simulink model "Model0_PWM_Base"  (R2021b)
settings: Solver=ode23s  StartTime=0.0  StopTime=20  MaxStep=1e-6  RelTol=1e-5  EnableMultiTasking=on
InitFcn:
  | L=5e-3
  | R=0.1
  | tau=10e-3
  | f_grid=50
  | Vpeak_d1=400*sqrt(2)/sqrt(3)
libraries: spsIGBTDiodeLib x6, spsControlledVoltageSourceLib x3, spsCurrentMeasurementLib x3, spsSeriesRLCBranchLib x3, spsVoltageMeasurementLib x3, spsDCVoltageSourceLib x2, spsGroundLib x1, simulink x1, spspowerguiLib x1
settings Model: Creator=Eduardo  LastModifiedBy=eprieto
settings SolverCC: ZeroCrossAlgorithm=Adaptive  AlgebraicLoopSolver=TrustRegion
settings DataIOCC: LimitDataPoints=on  SaveFormat=Array  SignalLoggingSaveFormat=ModelDataLogs  ReturnWorkspaceOutputs=off
settings OptimizationCC: LifeSpan=inf
settings DebuggingCC: SolverPrmCheckMsg=warning  MultiTaskDSMMsg=warning  MultiTaskCondExecSysMsg=none  StrictBusMsg=ErrorOnBusTreatedAsVector  SFUnexpectedBacktrackingDiag=warning  SFNoUnconditionalDefaultTransitionDiag=warning  SFExecutionAtInitializationDiag=none  SFMachineParentedDataDiag=warning  ArithmeticOperatorsInVariantConditions=warning
settings HardwareCC: ProdBitPerPointer=32  ProdBitPerSizeT=32  ProdBitPerPtrDiffT=32  ProdLargestAtomicFloat=None  ProdIntDivRoundTo=Undefined  ProdEndianess=Unspecified  ProdWordSize=32  ProdHWDeviceType=32-bit Generic
settings ModelReferenceCC: PropagateSignalLabelsOutOfModel=off
settings SFSimCC: SimUseLocalCustomCode=off  CustomCodeUndefinedFunction=UseInterfaceOnly
settings RTWCC: RTWUseLocalCustomCode=off
settings CodeAppCC: StateflowObjectComments=on
settings GRTTargetCC: TargetLangStandard=C89/C90 (ANSI)
settings ConfigComp: CovMetricSettings=dw  CovSaveCumulativeToWorkspaceVar=on  CovSaveSingleToWorkspaceVar=on  CovExternalEMLEnable=off
settings SimscapeCC: SimscapeNormalizeSystem=off

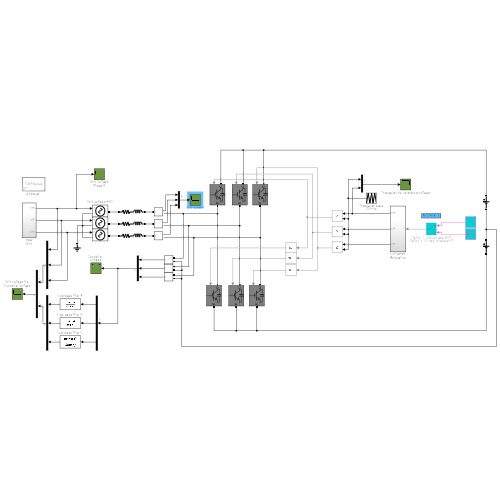
[thumbnail: Simulink's stored preview of the top-level diagram]
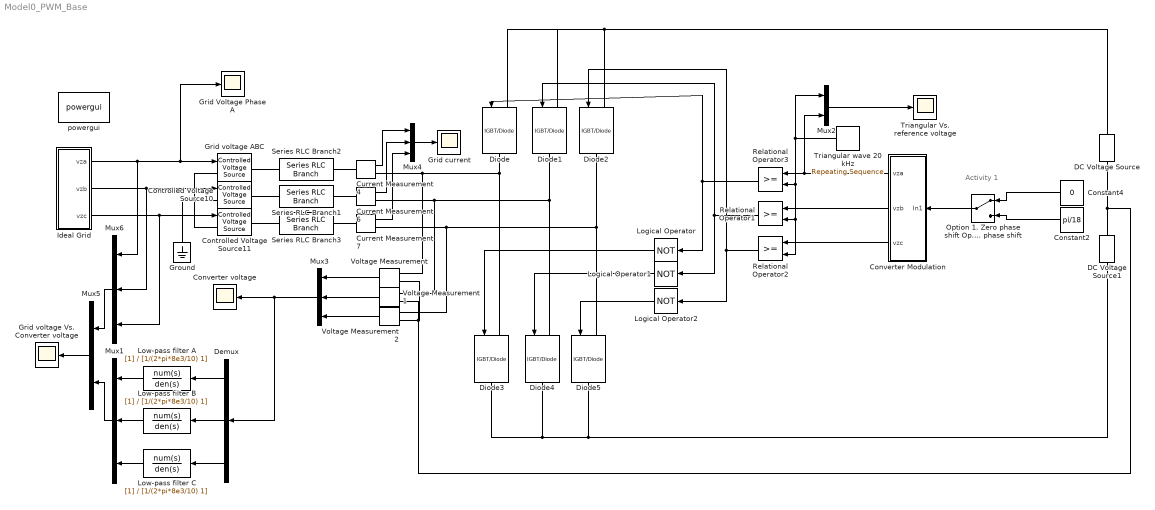
== system Model0_PWM_Base ==
  note: Activity 1
  Constant2 : Constant  Value=pi/18
  Constant4 : Constant  Value=0
  Controlled Voltage Source10 : spsControlledVoltageSourceLib/Controlled Voltage Source  Initialize=off  Source_Type=AC  Amplitude=0  Phase=0  Frequency=0  Measurements=None
  Controlled Voltage Source11 : spsControlledVoltageSourceLib/Controlled Voltage Source  Initialize=off  Source_Type=AC  Amplitude=0  Phase=0  Frequency=0  Measurements=None
  Converter Modulation : Subsystem
  Converter voltage : Scope
  Current Measurement4 : spsCurrentMeasurementLib/Current Measurement  PhasorSimulation=off  OutputType=Complex  PSBequivalent=0
  Current Measurement6 : spsCurrentMeasurementLib/Current Measurement  PhasorSimulation=off  OutputType=Complex  PSBequivalent=0
  Current Measurement7 : spsCurrentMeasurementLib/Current Measurement  PhasorSimulation=off  OutputType=Complex  PSBequivalent=0
  DC Voltage Source : spsDCVoltageSourceLib/DC Voltage Source  Amplitude=Vpeak_d1  Measurements=None
  DC Voltage Source1 : spsDCVoltageSourceLib/DC Voltage Source  Amplitude=Vpeak_d1  Measurements=None
  Demux : Demux  Outputs=3
  Diode{,1..5} (6 alike) : spsIGBTDiodeLib/IGBT//Diode  Ron=1e-3  Rs=1e5  Cs=inf  Measurements=off
  Grid Voltage Phase A : Scope
  Grid current : Scope
  Grid voltage ABC : spsControlledVoltageSourceLib/Controlled Voltage Source  Initialize=off  Source_Type=AC  Amplitude=0  Phase=0  Frequency=0  Measurements=None
  Grid voltage Vs. Converter voltage : Scope
  Ground : spsGroundLib/Ground  LConnTagsString=a
  Ideal Grid : Subsystem
  Logical Operator : Logic  Operator=NOT  AllPortsSameDT=off
  Logical Operator1 : Logic  Operator=NOT  AllPortsSameDT=off
  Logical Operator2 : Logic  Operator=NOT  AllPortsSameDT=off
  Low-pass filter A : TransferFcn  Denominator=[1/(2*pi*8e3/10) 1]
  Low-pass filter B : TransferFcn  Denominator=[1/(2*pi*8e3/10) 1]
  Low-pass filter C : TransferFcn  Denominator=[1/(2*pi*8e3/10) 1]
  Mux{1,3..4,6} (4 alike) : Mux  Inputs=3
  Mux2 : Mux  Inputs=2
  Mux5 : Mux  Inputs=2
  "Option 1. Zero phase shift Option 2. 20 deg. phase shift " : ManualSwitch
  Relational Operator1 : RelationalOperator  RndMeth=Nearest
  Relational Operator2 : RelationalOperator  RndMeth=Nearest
  Relational Operator3 : RelationalOperator  RndMeth=Nearest
  Series RLC Branch1 : spsSeriesRLCBranchLib/Series RLC Branch  LConnTagsString=__new0  RConnTagsString=__new0  BranchType=RL  Resistance=R  Inductance=L  SetiL0=off  InitialCurrent=0  Capacitance=0  Setx0=off  InitialVoltage=0  Measurements=None
  Series RLC Branch2 : spsSeriesRLCBranchLib/Series RLC Branch  LConnTagsString=__new0  RConnTagsString=__new0  BranchType=RL  Resistance=R  Inductance=L  SetiL0=off  InitialCurrent=0  Capacitance=0  Setx0=off  InitialVoltage=0  Measurements=None
  Series RLC Branch3 : spsSeriesRLCBranchLib/Series RLC Branch  LConnTagsString=__new0  RConnTagsString=__new0  BranchType=RL  Resistance=R  Inductance=L  SetiL0=off  InitialCurrent=0  Capacitance=0  Setx0=off  InitialVoltage=0  Measurements=None
  Triangular Vs. reference voltage : Scope
  Triangular wave 20 kHz : simulink/Sources/Repeating Sequence  rep_seq_t=[0 1/20e3 1/20e3*2]  rep_seq_y=[-Vpeak_d1 Vpeak_d1 -Vpeak_d1]
  Voltage Measurement : spsVoltageMeasurementLib/Voltage Measurement  PhasorSimulation=off  OutputType=Complex  PSBequivalent=0
  Voltage Measurement1 : spsVoltageMeasurementLib/Voltage Measurement  PhasorSimulation=off  OutputType=Complex  PSBequivalent=0
  Voltage Measurement2 : spsVoltageMeasurementLib/Voltage Measurement  PhasorSimulation=off  OutputType=Complex  PSBequivalent=0
  powergui : spspowerguiLib/powergui  Priority=1  SimulationMode=Continuous  SampleTime=50e-6  frequency=60  Iterations=50  frequencyindice=0  Pbase=100e6  ErrMax=1e-4  UnitsV=kV  UnitsW=MW  buscounter=0  FunctionMessages=off  echomessages=off  EnableUseOfTLC=off  CurrentSourceSwitches=off  DisableSnubberDevices=off  DisableRonSwitches=off  DisableVfSwitches=off  DisplayEquations=off  AutomaticDiscreteSolvers=off  SolverType=Tustin  Interpol=off  ExternalGateDelay=off  methode=off  Ts=0  x0status=blocks  SPID=off  SwTol=0  HookPort=off  NonlinearTolerance=1e-4  nMaxIteration=100  ContinueOnMaxIteration=off  RestoreLinks=warning  ResistiveCurrentMeasurement=off  Frange=[0:2:500]  Ylog=off  Xlog=on  ShowGrid=off  save=off  variable=ZData  structure=0  ZoomFFT=off  StartTime=0.0  cycles=1  DisplayStyle=1  fundamental=60  FreqAxis=off  MaxFrequency=1000  frequencyindicesteady=1  RmsSteady=1  display=off
  wires:
  Ideal Grid/1(vza) -> Mux6/1, Grid Voltage Phase A/1, Grid voltage ABC/1
  Ideal Grid/2(vzb) -> Mux6/2, Controlled Voltage Source10/1
  Ideal Grid/3(vzc) -> Mux6/3, Controlled Voltage Source11/1
  Current Measurement4/1 -> Mux4/1
  Current Measurement6/1 -> Mux4/2
  Current Measurement7/1 -> Mux4/3
  Converter Modulation/1(vza) -> Relational Operator3/1, Mux2/2
  Converter Modulation/2(vzb) -> Relational Operator1/1
  Converter Modulation/3(vzc) -> Relational Operator2/1
  Relational Operator3/1 -> Diode/1, Logical Operator/1
  Relational Operator1/1 -> Diode1/1, Logical Operator1/1
  Relational Operator2/1 -> Diode2/1, Logical Operator2/1
  Logical Operator/1 -> Diode3/1
  Mux2/1 -> Triangular Vs. reference voltage/1
  Voltage Measurement/1 -> Mux3/1
  Voltage Measurement1/1 -> Mux3/2
  Mux3/1 -> Converter voltage/1, Demux/1
  Mux4/1 -> Grid current/1
  Logical Operator1/1 -> Diode4/1
  Logical Operator2/1 -> Diode5/1
  Constant4/1 -> "Option 1. Zero phase shift Option 2. 20 deg. phase shift "/1
  Constant2/1 -> "Option 1. Zero phase shift Option 2. 20 deg. phase shift "/2
  "Option 1. Zero phase shift Option 2. 20 deg. phase shift "/1 -> Converter Modulation/1(In1)
  Voltage Measurement2/1 -> Mux3/3
  Triangular wave 20 kHz/1 -> Relational Operator3/2, Relational Operator2/2, Relational Operator1/2, Mux2/1
  Demux/1 -> Low-pass filter A/1
  Demux/2 -> Low-pass filter B/1
  Demux/3 -> Low-pass filter C/1
  Low-pass filter C/1 -> Mux1/3
  Low-pass filter B/1 -> Mux1/2
  Low-pass filter A/1 -> Mux1/1
  Mux5/1 -> Grid voltage Vs. Converter voltage/1
  Mux1/1 -> Mux5/2
  Mux6/1 -> Mux5/1
  connections:
  Grid voltage ABC/LConn1 -- Ground/LConn1 -- Controlled Voltage Source10/LConn1 -- Controlled Voltage Source11/LConn1
  Current Measurement6/RConn1 -- Voltage Measurement1/LConn1 -- Diode1/RConn1 -- Diode4/LConn1
  Current Measurement4/LConn1 -- Series RLC Branch2/RConn1
  Series RLC Branch2/LConn1 -- Grid voltage ABC/RConn1
  Current Measurement7/LConn1 -- Series RLC Branch3/RConn1
  Current Measurement6/LConn1 -- Series RLC Branch1/RConn1
  Series RLC Branch3/LConn1 -- Controlled Voltage Source11/RConn1
  Current Measurement4/RConn1 -- Voltage Measurement/LConn1 -- Diode3/LConn1 -- Diode/RConn1
  Series RLC Branch1/LConn1 -- Controlled Voltage Source10/RConn1
  Diode1/LConn1 -- Diode/LConn1 -- DC Voltage Source/RConn1 -- Diode2/LConn1
  Diode3/RConn1 -- DC Voltage Source1/LConn1 -- Diode5/RConn1 -- Diode4/RConn1
  Current Measurement7/RConn1 -- Voltage Measurement2/LConn1 -- Diode2/RConn1 -- Diode5/LConn1
  DC Voltage Source/LConn1 -- Voltage Measurement2/LConn2 -- Voltage Measurement/LConn2 -- Voltage Measurement1/LConn2 -- DC Voltage Source1/RConn1

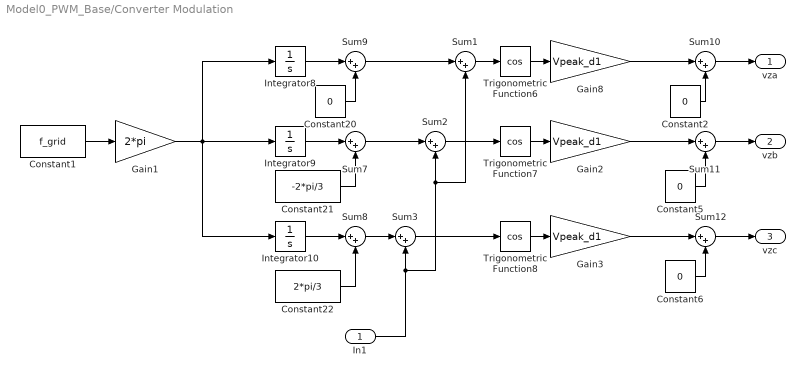
== system Model0_PWM_Base/Converter Modulation ==
  In1 : Inport
  Constant1 : Constant  Value=f_grid
  Constant{2,5..6,20} (4 alike) : Constant  Value=0
  Constant21 : Constant  Value=-2*pi/3
  Constant22 : Constant  Value=2*pi/3
  Gain1 : Gain  Gain=2*pi
  Gain2 : Gain  Gain=Vpeak_d1
  Gain3 : Gain  Gain=Vpeak_d1
  Gain8 : Gain  Gain=Vpeak_d1
  Integrator10 : Integrator
  Integrator8 : Integrator
  Integrator9 : Integrator
  Sum{1..3,7..12} (9 alike) : Sum  Inputs=|++
  Trigonometric Function6 : Trigonometry  Operator=cos
  Trigonometric Function7 : Trigonometry  Operator=cos
  Trigonometric Function8 : Trigonometry  Operator=cos
  vza : Outport
  vzb : Outport  Port=2
  vzc : Outport  Port=3
  wires:
  In1/1 -> Sum3/2, Sum2/2, Sum1/2
  Sum3/1 -> Trigonometric Function8/1
  Sum2/1 -> Trigonometric Function7/1
  Sum1/1 -> Trigonometric Function6/1
  Sum8/1 -> Sum3/1
  Integrator9/1 -> Sum7/1
  Trigonometric Function6/1 -> Gain8/1
  Constant20/1 -> Sum9/2
  Sum7/1 -> Sum2/1
  Integrator8/1 -> Sum9/1
  Constant21/1 -> Sum7/2
  Integrator10/1 -> Sum8/1
  Constant22/1 -> Sum8/2
  Sum9/1 -> Sum1/1
  Constant1/1 -> Gain1/1
  Trigonometric Function8/1 -> Gain3/1
  Trigonometric Function7/1 -> Gain2/1
  Gain1/1 -> Integrator10/1, Integrator8/1, Integrator9/1
  Gain8/1 -> Sum10/1
  Gain2/1 -> Sum11/1
  Gain3/1 -> Sum12/1
  Constant2/1 -> Sum10/2
  Constant5/1 -> Sum11/2
  Constant6/1 -> Sum12/2
  Sum10/1 -> vza/1
  Sum11/1 -> vzb/1
  Sum12/1 -> vzc/1

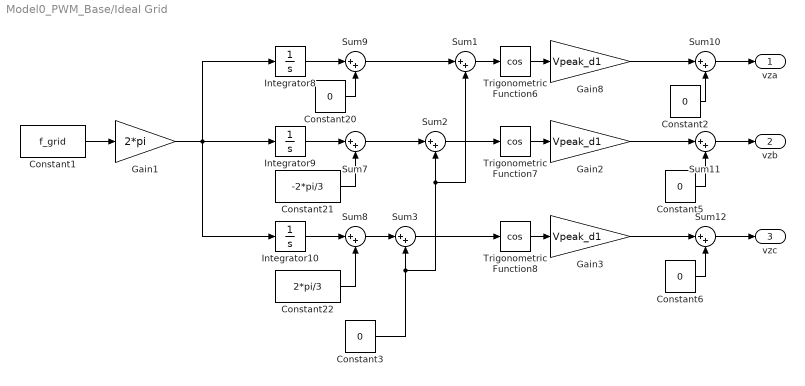
== system Model0_PWM_Base/Ideal Grid ==
  Constant1 : Constant  Value=f_grid
  Constant{2..3,5..6,20} (5 alike) : Constant  Value=0
  Constant21 : Constant  Value=-2*pi/3
  Constant22 : Constant  Value=2*pi/3
  Gain1 : Gain  Gain=2*pi
  Gain2 : Gain  Gain=Vpeak_d1
  Gain3 : Gain  Gain=Vpeak_d1
  Gain8 : Gain  Gain=Vpeak_d1
  Integrator10 : Integrator
  Integrator8 : Integrator
  Integrator9 : Integrator
  Sum{1..3,7..12} (9 alike) : Sum  Inputs=|++
  Trigonometric Function6 : Trigonometry  Operator=cos
  Trigonometric Function7 : Trigonometry  Operator=cos
  Trigonometric Function8 : Trigonometry  Operator=cos
  vza : Outport
  vzb : Outport  Port=2
  vzc : Outport  Port=3
  wires:
  Sum12/1 -> vzc/1
  Sum11/1 -> vzb/1
  Sum10/1 -> vza/1
  Constant6/1 -> Sum12/2
  Constant5/1 -> Sum11/2
  Constant2/1 -> Sum10/2
  Gain3/1 -> Sum12/1
  Gain2/1 -> Sum11/1
  Gain8/1 -> Sum10/1
  Gain1/1 -> Integrator9/1, Integrator8/1, Integrator10/1
  Trigonometric Function7/1 -> Gain2/1
  Trigonometric Function8/1 -> Gain3/1
  Constant1/1 -> Gain1/1
  Sum9/1 -> Sum1/1
  Constant22/1 -> Sum8/2
  Integrator10/1 -> Sum8/1
  Constant21/1 -> Sum7/2
  Integrator8/1 -> Sum9/1
  Sum7/1 -> Sum2/1
  Constant20/1 -> Sum9/2
  Trigonometric Function6/1 -> Gain8/1
  Integrator9/1 -> Sum7/1
  Sum8/1 -> Sum3/1
  Sum1/1 -> Trigonometric Function6/1
  Sum2/1 -> Trigonometric Function7/1
  Sum3/1 -> Trigonometric Function8/1
  Constant3/1 -> Sum1/2, Sum2/2, Sum3/2
